simulink model "CardioVascularSystem"  (R2021b)
settings: Solver=daessc  StartTime=0.0  StopTime=Tend  MaxStep=0.6  RelTol=1e-3  AbsTol=1e-3
undefined symbols (not defined in the file): EsL, EsR, PipL, PipR, R1, R2, R3_fix, R4, R5, R6, R7, R8, RL, RR, tc, ts
libraries: fl_lib x54, nesl_utility x23, ee_lib x4, SignalEditorBlockLib x1
settings Model: Creator=mnord  LastModifiedBy=mnord
settings SolverCC: ZeroCrossAlgorithm=Adaptive  AlgebraicLoopSolver=TrustRegion
settings DebuggingCC: MaxConsecutiveZCsMsg=warning  IgnoredZcDiagnostic=none  SymbolicDimsDataTypeCodeGenerationDiagnostic=none  SFMachineParentedDataDiag=warning
settings SFSimCC: CustomCodeUndefinedFunction=UseInterfaceOnly
settings SimscapeCC: SimscapeLogType=all  SimscapeLogSimulationStatistics=on  SimscapeLogDataHistory=10000

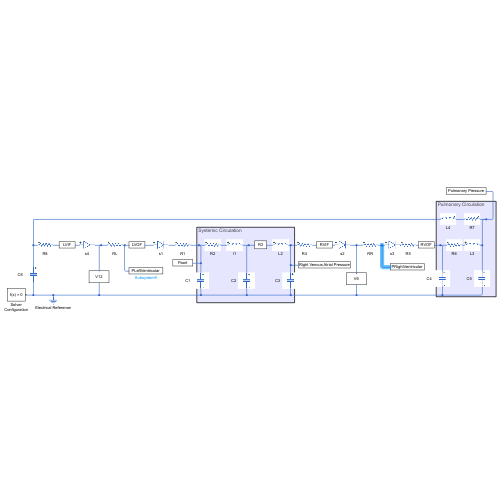
[thumbnail: Simulink's stored preview of the top-level diagram]
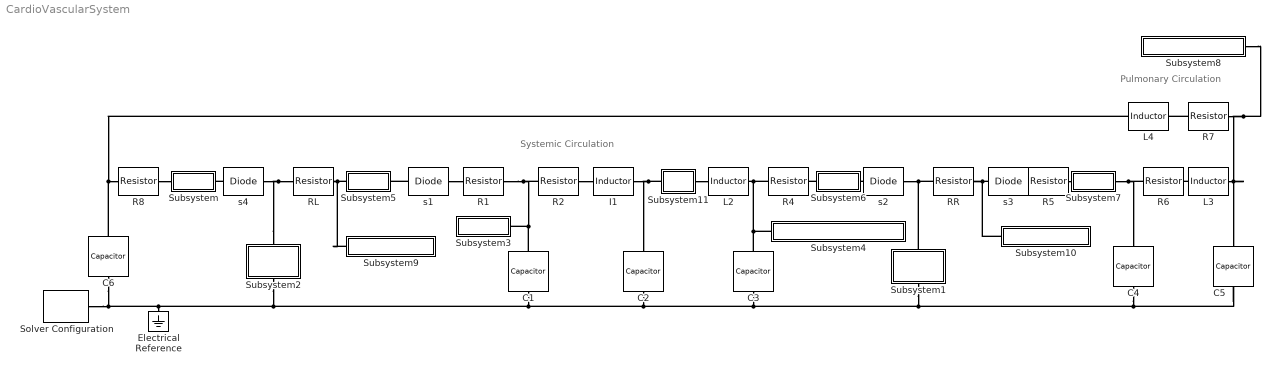
== system CardioVascularSystem ==
  note: Pulmonary Circulation
  note: Systemic Circulation
  C1 : fl_lib/Electrical/Electrical Elements/Capacitor  c=C1 F  r=capSerRes Ohm  g=0 1/Ohm  i_specify=off  i_priority=None  i=0 A  i_nominal_specify=off  i_nominal_unit=A  i_nominal_value=1  v_specify=off  v_priority=High  v=X10 V  v_nominal_specify=off  v_nominal_unit=V  v_nominal_value=1  vc_specify=on  vc_priority=High  vc=X10 V  vc_nominal_specify=off  vc_nominal_unit=V  vc_nominal_value=1
  C2 : fl_lib/Electrical/Electrical Elements/Capacitor  c=C2 F  r=capSerRes Ohm  g=0 1/Ohm  i_specify=off  i_priority=None  i=0 A  i_nominal_specify=off  i_nominal_unit=A  i_nominal_value=1  v_specify=off  v_priority=High  v=X30 V  v_nominal_specify=off  v_nominal_unit=V  v_nominal_value=1  vc_specify=on  vc_priority=High  vc=X30 V  vc_nominal_specify=off  vc_nominal_unit=V  vc_nominal_value=1
  C3 : fl_lib/Electrical/Electrical Elements/Capacitor  c=C3 F  r=capSerRes Ohm  g=0 1/Ohm  i_specify=off  i_priority=None  i=0 A  i_nominal_specify=off  i_nominal_unit=A  i_nominal_value=1  v_specify=off  v_priority=High  v=X50 V  v_nominal_specify=off  v_nominal_unit=V  v_nominal_value=1  vc_specify=on  vc_priority=High  vc=X50 V  vc_nominal_specify=off  vc_nominal_unit=V  vc_nominal_value=1
  C4 : fl_lib/Electrical/Electrical Elements/Capacitor  c=C4 F  r=capSerRes Ohm  g=0 1/Ohm  i_specify=off  i_priority=None  i=0 A  i_nominal_specify=off  i_nominal_unit=A  i_nominal_value=1  v_specify=off  v_priority=High  v=X70 V  v_nominal_specify=off  v_nominal_unit=V  v_nominal_value=1  vc_specify=on  vc_priority=High  vc=X70 V  vc_nominal_specify=off  vc_nominal_unit=V  vc_nominal_value=1
  C5 : fl_lib/Electrical/Electrical Elements/Capacitor  c=C5 F  r=capSerRes Ohm  g=0 1/Ohm  i_specify=off  i_priority=None  i=0 A  i_nominal_specify=off  i_nominal_unit=A  i_nominal_value=1  v_specify=off  v_priority=High  v=X90 V  v_nominal_specify=off  v_nominal_unit=V  v_nominal_value=1  vc_specify=on  vc_priority=High  vc=X90 V  vc_nominal_specify=off  vc_nominal_unit=V  vc_nominal_value=1
  C6 : fl_lib/Electrical/Electrical Elements/Capacitor  c=C6 F  r=capSerRes Ohm  g=0 1/Ohm  i_specify=off  i_priority=None  i=0 A  i_nominal_specify=off  i_nominal_unit=A  i_nominal_value=1  v_specify=off  v_priority=High  v=X110 V  v_nominal_specify=off  v_nominal_unit=V  v_nominal_value=1  vc_specify=on  vc_priority=High  vc=X110 V  vc_nominal_specify=off  vc_nominal_unit=V  vc_nominal_value=1
  Electrical Reference : fl_lib/Electrical/Electrical Elements/Electrical Reference
  I1 : ee_lib/Passive/Inductor  l=L1 H  L_tol=20  enable_L_tol=0  tol_distribution=1  nSigma=4  r=0 Ohm  g=1e-9 1/Ohm  enable_operating_limits=0  operating_limit_action=2  max_working_current=1 A  power_rating=1 W  enable_faults=0  fault_action=1  lambdaPercent=50  k_faulted=0.9999  turnsShort=0  openCct=0  groundShort=0  groundShortG=0 1/Ohm  tau_fault=1e-3 s  enable_temporal_fault=0  t_fault=1 s  enable_behavioral_fault=0  max_permissible_voltage=100 V  n_fail_on_voltage=1  max_permissible_current=1 A  t_fail_on_current=1 s  i_L_specify=on  i_L_priority=High  i_L=X20 A  i_L_nominal_specify=off  i_L_nominal_unit=A  i_L_nominal_value=1
  L2 : ee_lib/Passive/Inductor  l=L2 H  L_tol=20  enable_L_tol=0  tol_distribution=1  nSigma=4  r=0 Ohm  g=1e-9 1/Ohm  enable_operating_limits=0  operating_limit_action=2  max_working_current=1 A  power_rating=1 W  enable_faults=0  fault_action=1  lambdaPercent=50  k_faulted=0.9999  turnsShort=0  openCct=0  groundShort=0  groundShortG=0 1/Ohm  tau_fault=1e-3 s  enable_temporal_fault=0  t_fault=1 s  enable_behavioral_fault=0  max_permissible_voltage=100 V  n_fail_on_voltage=1  max_permissible_current=1 A  t_fail_on_current=1 s  i_L_specify=on  i_L_priority=High  i_L=X40 A  i_L_nominal_specify=off  i_L_nominal_unit=A  i_L_nominal_value=1
  L3 : ee_lib/Passive/Inductor  l=L3 H  L_tol=20  enable_L_tol=0  tol_distribution=1  nSigma=4  r=0 Ohm  g=1e-9 1/Ohm  enable_operating_limits=0  operating_limit_action=2  max_working_current=1 A  power_rating=1 W  enable_faults=0  fault_action=1  lambdaPercent=50  k_faulted=0.9999  turnsShort=0  openCct=0  groundShort=0  groundShortG=0 1/Ohm  tau_fault=1e-3 s  enable_temporal_fault=0  t_fault=1 s  enable_behavioral_fault=0  max_permissible_voltage=100 V  n_fail_on_voltage=1  max_permissible_current=1 A  t_fail_on_current=1 s  i_L_specify=on  i_L_priority=High  i_L=X80 A  i_L_nominal_specify=off  i_L_nominal_unit=A  i_L_nominal_value=1
  L4 : ee_lib/Passive/Inductor  l=L4 H  L_tol=20  enable_L_tol=0  tol_distribution=1  nSigma=4  r=0 Ohm  g=1e-9 1/Ohm  enable_operating_limits=0  operating_limit_action=2  max_working_current=1 A  power_rating=1 W  enable_faults=0  fault_action=1  lambdaPercent=50  k_faulted=0.9999  turnsShort=0  openCct=0  groundShort=0  groundShortG=0 1/Ohm  tau_fault=1e-3 s  enable_temporal_fault=0  t_fault=1 s  enable_behavioral_fault=0  max_permissible_voltage=100 V  n_fail_on_voltage=1  max_permissible_current=1 A  t_fail_on_current=1 s  i_L_specify=on  i_L_priority=High  i_L=X100 A  i_L_nominal_specify=off  i_L_nominal_unit=A  i_L_nominal_value=1
  R1 : fl_lib/Electrical/Electrical Elements/Resistor  R=R1 Ohm  i_specify=off  i_priority=None  i=0 A  i_nominal_specify=off  i_nominal_unit=A  i_nominal_value=1  v_specify=off  v_priority=None  v=0 V  v_nominal_specify=off  v_nominal_unit=V  v_nominal_value=1
  R2 : fl_lib/Electrical/Electrical Elements/Resistor  R=R2 Ohm  i_specify=off  i_priority=None  i=0 A  i_nominal_specify=off  i_nominal_unit=A  i_nominal_value=1  v_specify=off  v_priority=None  v=0 V  v_nominal_specify=off  v_nominal_unit=V  v_nominal_value=1
  R4 : fl_lib/Electrical/Electrical Elements/Resistor  R=R4 Ohm  i_specify=off  i_priority=None  i=0 A  i_nominal_specify=off  i_nominal_unit=A  i_nominal_value=1  v_specify=off  v_priority=None  v=0 V  v_nominal_specify=off  v_nominal_unit=V  v_nominal_value=1
  R5 : fl_lib/Electrical/Electrical Elements/Resistor  R=R5 Ohm  i_specify=off  i_priority=None  i=0 A  i_nominal_specify=off  i_nominal_unit=A  i_nominal_value=1  v_specify=off  v_priority=None  v=0 V  v_nominal_specify=off  v_nominal_unit=V  v_nominal_value=1
  R6 : fl_lib/Electrical/Electrical Elements/Resistor  R=R6 Ohm  i_specify=off  i_priority=None  i=0 A  i_nominal_specify=off  i_nominal_unit=A  i_nominal_value=1  v_specify=off  v_priority=None  v=0 V  v_nominal_specify=off  v_nominal_unit=V  v_nominal_value=1
  R7 : fl_lib/Electrical/Electrical Elements/Resistor  R=R7 Ohm  i_specify=off  i_priority=None  i=0 A  i_nominal_specify=off  i_nominal_unit=A  i_nominal_value=1  v_specify=off  v_priority=None  v=0 V  v_nominal_specify=off  v_nominal_unit=V  v_nominal_value=1
  R8 : fl_lib/Electrical/Electrical Elements/Resistor  R=R8 Ohm  i_specify=off  i_priority=None  i=0 A  i_nominal_specify=off  i_nominal_unit=A  i_nominal_value=1  v_specify=off  v_priority=None  v=0 V  v_nominal_specify=off  v_nominal_unit=V  v_nominal_value=1
  RL : fl_lib/Electrical/Electrical Elements/Resistor  R=RL Ohm  i_specify=off  i_priority=None  i=0 A  i_nominal_specify=off  i_nominal_unit=A  i_nominal_value=1  v_specify=off  v_priority=None  v=0 V  v_nominal_specify=off  v_nominal_unit=V  v_nominal_value=1
  RR : fl_lib/Electrical/Electrical Elements/Resistor  R=RR Ohm  i_specify=off  i_priority=None  i=0 A  i_nominal_specify=off  i_nominal_unit=A  i_nominal_value=1  v_specify=off  v_priority=None  v=0 V  v_nominal_specify=off  v_nominal_unit=V  v_nominal_value=1
  Solver Configuration : nesl_utility/Solver Configuration  PhysicalDomain=network_engine_domain  SubClassName=solver  LeftPortType=input  RightPortType=generic  Tones=[]  Harmonics=[]  SimulateNoise=off  Profile=off  UseLocalSampling=off  EnableSwitchedLinearOptims=on  FrequencyDomain=off  UseCCode=off  RelTol=0.001  AbsTol=1e-06  MinStep=1e-09  ToWorkspace=off  RevertToSquareIcSolve=off  NumHomotopyIterations=100  PhasorMode=off  PhasorModeNumHarmonics=1  DoDC=off  ResidualTolerance=1e-09  UseLocalSolver=off  LocalSolverChoice=NE_BACKWARD_EULER_ADVANCER  LocalSolverSampleTime=0.001  DoFixedCost=off  MaxNonlinIter=3  MaxModeIter=2  ComputeImpulses=off  ImpulseIterations=2  LinearAlgebra=auto  EquationFormulation=NE_TIME_EF  DelaysMemoryBudget=1024  AutomaticFiltering=on  FilteringTimeConstant=0.001  PartitionStorageMethod=AS_NEEDED  PartitionMemoryBudget=1024  PartitionMethod=ROBUST
      settings: SourceProductBaseCode=PW,SS
  Subsystem : Subsystem
      mask Display: disp('LVIF')
  Subsystem1 : Subsystem
      mask Display: disp('V6')
  Subsystem10 : Subsystem
      mask Display: disp('PRightVentricular')
  Subsystem11 : Subsystem
      mask Display: disp('R3')
  Subsystem2 : Subsystem
      mask Display: disp('V12')
  Subsystem3 : Subsystem
      mask Display: disp('Paort')
  Subsystem4 : Subsystem
      mask Display: disp('Right Venous Atrial Pressure')
  Subsystem5 : Subsystem
      mask Display: disp('LVOF')
  Subsystem6 : Subsystem
      mask Display: disp('RVIF')
  Subsystem7 : Subsystem
      mask Display: disp('RVOF')
  Subsystem8 : Subsystem
      mask Display: disp('Pulmonary Pressure')
  Subsystem9 : Subsystem
      mask Display: disp('PLeftVentricular')
  s{1..4} (4 alike) : fl_lib/Electrical/Electrical Elements/Diode  Vf=FwVolt V  Ron=onRes Ohm  Goff=1e-8 1/Ohm  i_specify=off  i_priority=None  i=0 A  i_nominal_specify=off  i_nominal_unit=A  i_nominal_value=1  v_specify=off  v_priority=None  v=0 V  v_nominal_specify=off  v_nominal_unit=V  v_nominal_value=1
  connections:
  C6/LConn1 -- R8/LConn1 -- L4/RConn1
  Subsystem11/RConn1 -- L2/LConn1
  I1/RConn1 -- Subsystem11/LConn1 -- C2/LConn1
  R4/LConn1 -- C3/LConn1 -- Subsystem4/LConn1 -- L2/RConn1
  L3/LConn1 -- R6/RConn1
  L3/RConn1 -- Subsystem8/LConn1 -- R7/LConn1 -- C5/LConn1
  R7/RConn1 -- L4/LConn1
  R8/RConn1 -- Subsystem/LConn1
  s4/LConn1 -- Subsystem/RConn1
  Subsystem3/LConn1 -- R2/LConn1 -- R1/RConn1 -- C1/LConn1
  Subsystem6/LConn1 -- R4/RConn1
  C6/RConn1 -- Solver Configuration/RConn1 -- Electrical Reference/LConn1 -- Subsystem2/RConn1 -- C5/RConn1 -- C4/RConn1 -- Subsystem1/RConn1 -- C3/RConn1 -- C2/RConn1 -- C1/RConn1
  RR/LConn1 -- Subsystem1/LConn1 -- s2/RConn1
  Subsystem2/LConn1 -- s4/RConn1 -- RL/LConn1
  s3/LConn1 -- Subsystem10/LConn1 -- RR/RConn1
  s3/RConn1 -- R5/LConn1
  R6/LConn1 -- C4/LConn1 -- Subsystem7/RConn1
  Subsystem5/LConn1 -- Subsystem9/LConn1 -- RL/RConn1
  s1/RConn1 -- R1/LConn1
  s2/LConn1 -- Subsystem6/RConn1
  R5/RConn1 -- Subsystem7/LConn1
  s1/LConn1 -- Subsystem5/RConn1
  R2/RConn1 -- I1/LConn1

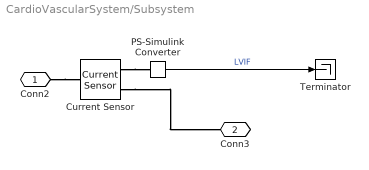
== system CardioVascularSystem/Subsystem ==
  Current Sensor : fl_lib/Electrical/Electrical Sensors/Current Sensor
  PS-Simulink Converter : nesl_utility/PS-Simulink Converter  PhysicalDomain=network_engine_domain  SubClassName=ps_output  LeftPortType=input  RightPortType=output  PseudoPeriodic=off  Frequencies=[]  Unit=inherit  AffineConversion=off
      settings: SourceProductBaseCode=PW,SS
  Terminator : Terminator
  Conn2 : PMIOPort  Side=Left
  Conn3 : PMIOPort  Port=2  Side=Right
  wires:
  PS-Simulink Converter/1 -> Terminator/1  "LVIF"
  connections:
  Conn2/RConn1 -- Current Sensor/LConn1
  Current Sensor/RConn2 -- Conn3/RConn1
  Current Sensor/RConn1 -- PS-Simulink Converter/LConn1

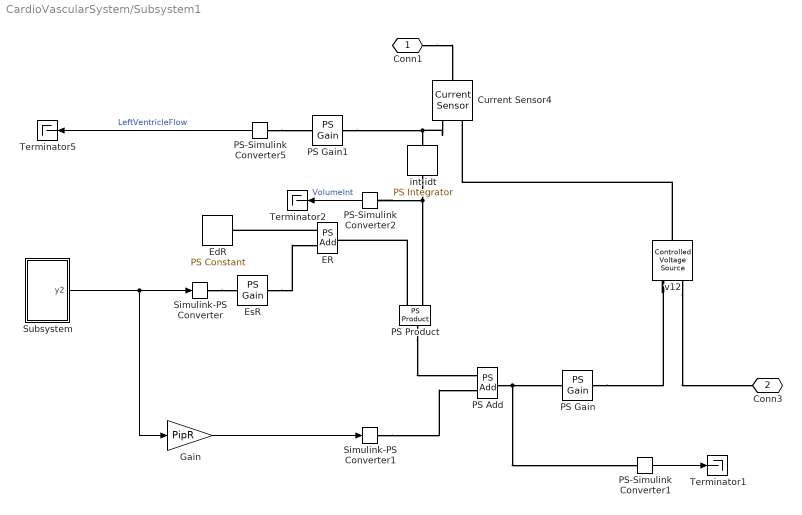
== system CardioVascularSystem/Subsystem1 ==
  Current Sensor4 : fl_lib/Electrical/Electrical Sensors/Current Sensor
  ER : fl_lib/Physical Signals/Functions/PS Add
  EdR : fl_lib/Physical Signals/Sources/PS Constant  constant=EdR
  EsR : fl_lib/Physical Signals/Functions/PS Gain  gain=EsR
  Gain : Gain  Gain=PipR
  PS Add : fl_lib/Physical Signals/Functions/PS Add
  PS Gain : fl_lib/Physical Signals/Functions/PS Gain  gain=1 V/s/A
  PS Gain1 : fl_lib/Physical Signals/Functions/PS Gain  gain=-1
  PS Product : fl_lib/Physical Signals/Functions/PS Product
  PS-Simulink Converter1 : nesl_utility/PS-Simulink Converter  PhysicalDomain=network_engine_domain  SubClassName=ps_output  LeftPortType=input  RightPortType=output  PseudoPeriodic=off  Frequencies=[]  Unit=inherit  AffineConversion=off
      settings: SourceProductBaseCode=PW,SS
  PS-Simulink Converter2 : nesl_utility/PS-Simulink Converter  PhysicalDomain=network_engine_domain  SubClassName=ps_output  LeftPortType=input  RightPortType=output  PseudoPeriodic=off  Frequencies=[]  Unit=inherit  AffineConversion=off
      settings: SourceProductBaseCode=PW,SS
  PS-Simulink Converter5 : nesl_utility/PS-Simulink Converter  PhysicalDomain=network_engine_domain  SubClassName=ps_output  LeftPortType=input  RightPortType=output  PseudoPeriodic=off  Frequencies=[]  Unit=inherit  AffineConversion=off
      settings: SourceProductBaseCode=PW,SS
  Simulink-PS Converter : nesl_utility/Simulink-PS Converter  PhysicalDomain=network_engine_domain  SubClassName=ps_input  LeftPortType=input  RightPortType=output  PseudoPeriodic=off  Frequencies=[]  NoiseDistribution=none  NoiseParameters=[]  Unit=1  AffineConversion=off  FilteringAndDerivatives=provide  SimscapeFilterOrder=1  InputFilterTimeConstant=0.001  UdotUserProvided=0
      settings: SourceProductBaseCode=PW,SS
  Simulink-PS Converter1 : nesl_utility/Simulink-PS Converter  PhysicalDomain=network_engine_domain  SubClassName=ps_input  LeftPortType=input  RightPortType=output  PseudoPeriodic=off  Frequencies=[]  NoiseDistribution=none  NoiseParameters=[]  Unit=A*s  AffineConversion=off  FilteringAndDerivatives=provide  SimscapeFilterOrder=1  InputFilterTimeConstant=0.001  UdotUserProvided=0
      settings: SourceProductBaseCode=PW,SS
  Subsystem : Subsystem
  Terminator1 : Terminator
  Terminator2 : Terminator
  Terminator5 : Terminator
  int idt : fl_lib/Physical Signals/Linear Operators/PS Integrator  reset_method=foundation.enum.IntegratorResetSpec.None  initial_condition_spec=foundation.enum.IntegratorICSpec.Internal  x0=X60 A*s
      settings: SourceProductBaseCode=SS
  v12 : fl_lib/Electrical/Electrical Sources/Controlled Voltage Source
  Conn1 : PMIOPort  Side=Left
  Conn3 : PMIOPort  Port=2  Side=Right
  wires:
  PS-Simulink Converter1/1 -> Terminator1/1
  Gain/1 -> Simulink-PS Converter1/1
  PS-Simulink Converter2/1 -> Terminator2/1  "VolumeInt"
  Subsystem/1(y2) -> Gain/1, Simulink-PS Converter/1
  PS-Simulink Converter5/1 -> Terminator5/1  "LeftVentricleFlow"
  connections:
  PS Add/RConn1 -- PS-Simulink Converter1/LConn1 -- PS Gain/LConn1
  PS-Simulink Converter2/LConn1 -- PS Product/LConn1 -- int idt/RConn1
  PS Product/RConn1 -- PS Add/LConn1
  v12/LConn1 -- Current Sensor4/RConn2
  ER/LConn1 -- EdR/RConn1
  Simulink-PS Converter1/RConn1 -- PS Add/LConn2
  EsR/RConn1 -- ER/LConn2
  PS Product/LConn2 -- ER/RConn1
  v12/RConn2 -- Conn3/RConn1
  Conn1/RConn1 -- Current Sensor4/LConn1
  Current Sensor4/RConn1 -- PS Gain1/LConn1 -- int idt/LConn1
  Simulink-PS Converter/RConn1 -- EsR/LConn1
  PS Gain/RConn1 -- v12/RConn1
  PS-Simulink Converter5/LConn1 -- PS Gain1/RConn1

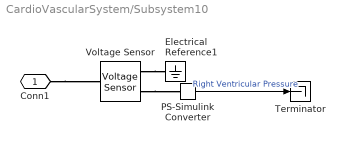
== system CardioVascularSystem/Subsystem10 ==
  Electrical Reference1 : fl_lib/Electrical/Electrical Elements/Electrical Reference
  PS-Simulink Converter : nesl_utility/PS-Simulink Converter  PhysicalDomain=network_engine_domain  SubClassName=ps_output  LeftPortType=input  RightPortType=output  PseudoPeriodic=off  Frequencies=[]  Unit=inherit  AffineConversion=off
      settings: SourceProductBaseCode=PW,SS
  Terminator : Terminator
  Voltage Sensor : fl_lib/Electrical/Electrical Sensors/Voltage Sensor
  Conn1 : PMIOPort  Side=Left
  wires:
  PS-Simulink Converter/1 -> Terminator/1  "Right Ventricular Pressure"
  connections:
  Conn1/RConn1 -- Voltage Sensor/LConn1
  Voltage Sensor/RConn2 -- Electrical Reference1/LConn1
  Voltage Sensor/RConn1 -- PS-Simulink Converter/LConn1

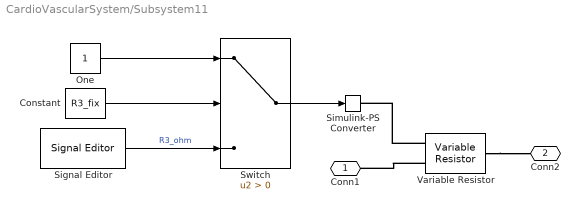
== system CardioVascularSystem/Subsystem11 ==
  Constant : Constant  Value=R3_fix
  One : Constant  OutDataTypeStr=Inherit: Inherit via back propagation
  Signal Editor : SignalEditorBlockLib/Signal Editor  FileName=R3_Values.mat  ActiveScenario=Scenario  ActiveSignal=Signal 1  IsBus=off  OutputBusObjectStr=Bus: BusObject  SampleTime=0  Interpolate=off  ZeroCross=off  OutputAfterFinalValue=Holding final value  Unit=inherit  PreserveSignalName=on
  Simulink-PS Converter : nesl_utility/Simulink-PS Converter  PhysicalDomain=network_engine_domain  SubClassName=ps_input  LeftPortType=input  RightPortType=output  PseudoPeriodic=off  Frequencies=[]  NoiseDistribution=none  NoiseParameters=[]  Unit=1  AffineConversion=off  FilteringAndDerivatives=filter  SimscapeFilterOrder=1  InputFilterTimeConstant=0.1  UdotUserProvided=0
      settings: SourceProductBaseCode=PW,SS
  Switch : Switch  Criteria=u2 > Threshold
  Variable Resistor : fl_lib/Electrical/Electrical Elements/Variable Resistor  Rmin=0 Ohm  i_specify=off  i_priority=None  i=0 A  i_nominal_specify=off  i_nominal_unit=A  i_nominal_value=1  v_specify=off  v_priority=None  v=0 V  v_nominal_specify=off  v_nominal_unit=V  v_nominal_value=1
  Conn1 : PMIOPort  Side=Left
  Conn2 : PMIOPort  Port=2  Side=Right
  wires:
  Signal Editor/1 -> Switch/3  "R3_ohm"
  One/1 -> Switch/1
  Constant/1 -> Switch/2
  Switch/1 -> Simulink-PS Converter/1
  connections:
  Variable Resistor/LConn1 -- Simulink-PS Converter/RConn1
  Variable Resistor/LConn2 -- Conn1/RConn1
  Variable Resistor/RConn1 -- Conn2/RConn1

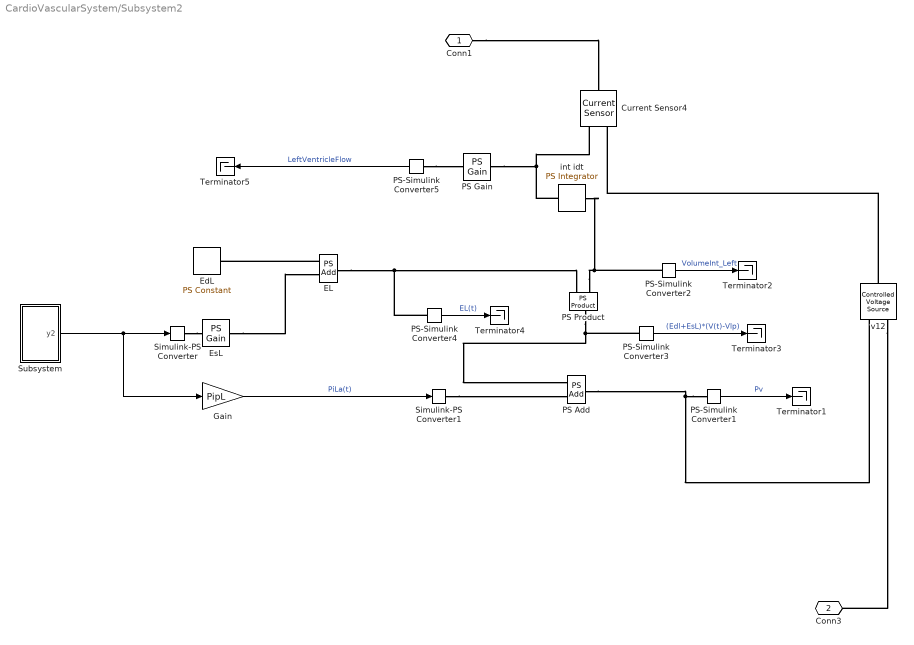
== system CardioVascularSystem/Subsystem2 ==
  Current Sensor4 : fl_lib/Electrical/Electrical Sensors/Current Sensor
  EL : fl_lib/Physical Signals/Functions/PS Add
  EdL : fl_lib/Physical Signals/Sources/PS Constant  constant=EdL V/A/s
  EsL : fl_lib/Physical Signals/Functions/PS Gain  gain=EsL
  Gain : Gain  Gain=PipL
  PS Add : fl_lib/Physical Signals/Functions/PS Add
  PS Gain : fl_lib/Physical Signals/Functions/PS Gain  gain=-1
  PS Product : fl_lib/Physical Signals/Functions/PS Product
  PS-Simulink Converter{1..5} (5 alike) : nesl_utility/PS-Simulink Converter  PhysicalDomain=network_engine_domain  SubClassName=ps_output  LeftPortType=input  RightPortType=output  PseudoPeriodic=off  Frequencies=[]  Unit=inherit  AffineConversion=off
      settings: SourceProductBaseCode=PW,SS
  Simulink-PS Converter : nesl_utility/Simulink-PS Converter  PhysicalDomain=network_engine_domain  SubClassName=ps_input  LeftPortType=input  RightPortType=output  PseudoPeriodic=off  Frequencies=[]  NoiseDistribution=none  NoiseParameters=[]  Unit=V/A/s  AffineConversion=off  FilteringAndDerivatives=provide  SimscapeFilterOrder=1  InputFilterTimeConstant=0.001  UdotUserProvided=0
      settings: SourceProductBaseCode=PW,SS
  Simulink-PS Converter1 : nesl_utility/Simulink-PS Converter  PhysicalDomain=network_engine_domain  SubClassName=ps_input  LeftPortType=input  RightPortType=output  PseudoPeriodic=off  Frequencies=[]  NoiseDistribution=none  NoiseParameters=[]  Unit=V  AffineConversion=off  FilteringAndDerivatives=provide  SimscapeFilterOrder=1  InputFilterTimeConstant=0.001  UdotUserProvided=0
      settings: SourceProductBaseCode=PW,SS
  Subsystem : Subsystem
  Terminator{1..5} (5 alike) : Terminator
  int idt : fl_lib/Physical Signals/Linear Operators/PS Integrator  reset_method=foundation.enum.IntegratorResetSpec.None  initial_condition_spec=foundation.enum.IntegratorICSpec.Internal  x0=X120 A*s
      settings: SourceProductBaseCode=SS
  v12 : fl_lib/Electrical/Electrical Sources/Controlled Voltage Source
  Conn1 : PMIOPort  Side=Left
  Conn3 : PMIOPort  Port=2  Side=Right
  wires:
  Gain/1 -> Simulink-PS Converter1/1  "PiLa(t)"
  Subsystem/1(y2) -> Gain/1, Simulink-PS Converter/1
  PS-Simulink Converter1/1 -> Terminator1/1  "Pv"
  PS-Simulink Converter2/1 -> Terminator2/1  "VolumeInt_Left"
  PS-Simulink Converter3/1 -> Terminator3/1  "(Edl+EsL)*(V(t)-Vlp)"
  PS-Simulink Converter4/1 -> Terminator4/1  "EL(t)"
  PS-Simulink Converter5/1 -> Terminator5/1  "LeftVentricleFlow"
  connections:
  PS Product/LConn1 -- int idt/RConn1 -- PS-Simulink Converter2/LConn1
  EL/LConn1 -- EdL/RConn1
  EsL/RConn1 -- EL/LConn2
  Simulink-PS Converter1/RConn1 -- PS Add/LConn2
  Simulink-PS Converter/RConn1 -- EsL/LConn1
  v12/RConn2 -- Conn3/RConn1
  int idt/LConn1 -- PS Gain/LConn1 -- Current Sensor4/RConn1
  Conn1/RConn1 -- Current Sensor4/LConn1
  EL/RConn1 -- PS-Simulink Converter4/LConn1 -- PS Product/LConn2
  PS-Simulink Converter1/LConn1 -- v12/RConn1 -- PS Add/RConn1
  v12/LConn1 -- Current Sensor4/RConn2
  PS Product/RConn1 -- PS Add/LConn1 -- PS-Simulink Converter3/LConn1
  PS-Simulink Converter5/LConn1 -- PS Gain/RConn1

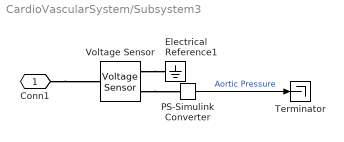
== system CardioVascularSystem/Subsystem3 ==
  Electrical Reference1 : fl_lib/Electrical/Electrical Elements/Electrical Reference
  PS-Simulink Converter : nesl_utility/PS-Simulink Converter  PhysicalDomain=network_engine_domain  SubClassName=ps_output  LeftPortType=input  RightPortType=output  PseudoPeriodic=off  Frequencies=[]  Unit=inherit  AffineConversion=off
      settings: SourceProductBaseCode=PW,SS
  Terminator : Terminator
  Voltage Sensor : fl_lib/Electrical/Electrical Sensors/Voltage Sensor
  Conn1 : PMIOPort  Side=Left
  wires:
  PS-Simulink Converter/1 -> Terminator/1  "Aortic Pressure"
  connections:
  Voltage Sensor/RConn1 -- PS-Simulink Converter/LConn1
  Voltage Sensor/RConn2 -- Electrical Reference1/LConn1
  Conn1/RConn1 -- Voltage Sensor/LConn1

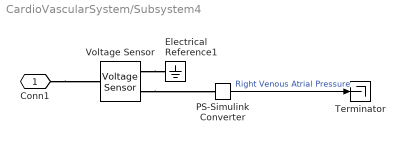
== system CardioVascularSystem/Subsystem4 ==
  Electrical Reference1 : fl_lib/Electrical/Electrical Elements/Electrical Reference
  PS-Simulink Converter : nesl_utility/PS-Simulink Converter  PhysicalDomain=network_engine_domain  SubClassName=ps_output  LeftPortType=input  RightPortType=output  PseudoPeriodic=off  Frequencies=[]  Unit=inherit  AffineConversion=off
      settings: SourceProductBaseCode=PW,SS
  Terminator : Terminator
  Voltage Sensor : fl_lib/Electrical/Electrical Sensors/Voltage Sensor
  Conn1 : PMIOPort  Side=Left
  wires:
  PS-Simulink Converter/1 -> Terminator/1  "Right Venous Atrial Pressure"
  connections:
  Conn1/RConn1 -- Voltage Sensor/LConn1
  Voltage Sensor/RConn2 -- Electrical Reference1/LConn1
  Voltage Sensor/RConn1 -- PS-Simulink Converter/LConn1

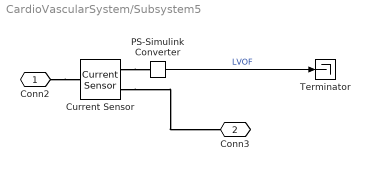
== system CardioVascularSystem/Subsystem5 ==
  Current Sensor : fl_lib/Electrical/Electrical Sensors/Current Sensor
  PS-Simulink Converter : nesl_utility/PS-Simulink Converter  PhysicalDomain=network_engine_domain  SubClassName=ps_output  LeftPortType=input  RightPortType=output  PseudoPeriodic=off  Frequencies=[]  Unit=inherit  AffineConversion=off
      settings: SourceProductBaseCode=PW,SS
  Terminator : Terminator
  Conn2 : PMIOPort  Side=Left
  Conn3 : PMIOPort  Port=2  Side=Right
  wires:
  PS-Simulink Converter/1 -> Terminator/1  "LVOF"
  connections:
  Conn2/RConn1 -- Current Sensor/LConn1
  Current Sensor/RConn2 -- Conn3/RConn1
  Current Sensor/RConn1 -- PS-Simulink Converter/LConn1

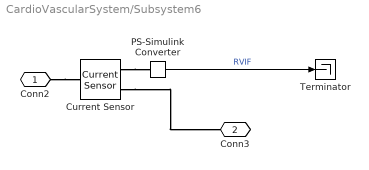
== system CardioVascularSystem/Subsystem6 ==
  Current Sensor : fl_lib/Electrical/Electrical Sensors/Current Sensor
  PS-Simulink Converter : nesl_utility/PS-Simulink Converter  PhysicalDomain=network_engine_domain  SubClassName=ps_output  LeftPortType=input  RightPortType=output  PseudoPeriodic=off  Frequencies=[]  Unit=inherit  AffineConversion=off
      settings: SourceProductBaseCode=PW,SS
  Terminator : Terminator
  Conn2 : PMIOPort  Side=Left
  Conn3 : PMIOPort  Port=2  Side=Right
  wires:
  PS-Simulink Converter/1 -> Terminator/1  "RVIF"
  connections:
  Current Sensor/RConn1 -- PS-Simulink Converter/LConn1
  Current Sensor/RConn2 -- Conn3/RConn1
  Conn2/RConn1 -- Current Sensor/LConn1

== system CardioVascularSystem/Subsystem7 ==
  Current Sensor : fl_lib/Electrical/Electrical Sensors/Current Sensor
  PS-Simulink Converter : nesl_utility/PS-Simulink Converter  PhysicalDomain=network_engine_domain  SubClassName=ps_output  LeftPortType=input  RightPortType=output  PseudoPeriodic=off  Frequencies=[]  Unit=inherit  AffineConversion=off
      settings: SourceProductBaseCode=PW,SS
  Terminator : Terminator
  Conn2 : PMIOPort  Side=Left
  Conn3 : PMIOPort  Port=2  Side=Right
  wires:
  PS-Simulink Converter/1 -> Terminator/1  "RVOF"
  connections:
  Conn2/RConn1 -- Current Sensor/LConn1
  Current Sensor/RConn2 -- Conn3/RConn1
  Current Sensor/RConn1 -- PS-Simulink Converter/LConn1

== system CardioVascularSystem/Subsystem8 ==
  Electrical Reference1 : fl_lib/Electrical/Electrical Elements/Electrical Reference
  PS-Simulink Converter : nesl_utility/PS-Simulink Converter  PhysicalDomain=network_engine_domain  SubClassName=ps_output  LeftPortType=input  RightPortType=output  PseudoPeriodic=off  Frequencies=[]  Unit=inherit  AffineConversion=off
      settings: SourceProductBaseCode=PW,SS
  Terminator : Terminator
  Voltage Sensor : fl_lib/Electrical/Electrical Sensors/Voltage Sensor
  Conn1 : PMIOPort  Side=Left
  wires:
  PS-Simulink Converter/1 -> Terminator/1  "Pulmonary Pressure"
  connections:
  Conn1/RConn1 -- Voltage Sensor/LConn1
  Voltage Sensor/RConn2 -- Electrical Reference1/LConn1
  Voltage Sensor/RConn1 -- PS-Simulink Converter/LConn1

== system CardioVascularSystem/Subsystem9 ==
  Electrical Reference1 : fl_lib/Electrical/Electrical Elements/Electrical Reference
  PS-Simulink Converter : nesl_utility/PS-Simulink Converter  PhysicalDomain=network_engine_domain  SubClassName=ps_output  LeftPortType=input  RightPortType=output  PseudoPeriodic=off  Frequencies=[]  Unit=inherit  AffineConversion=off
      settings: SourceProductBaseCode=PW,SS
  Terminator : Terminator
  Voltage Sensor : fl_lib/Electrical/Electrical Sensors/Voltage Sensor
  Conn1 : PMIOPort  Side=Left
  wires:
  PS-Simulink Converter/1 -> Terminator/1  "Left Ventricular Pressure"
  connections:
  Conn1/RConn1 -- Voltage Sensor/LConn1
  Voltage Sensor/RConn2 -- Electrical Reference1/LConn1
  Voltage Sensor/RConn1 -- PS-Simulink Converter/LConn1

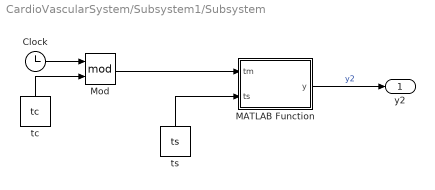
== system CardioVascularSystem/Subsystem1/Subsystem ==
  Clock : Clock
  MATLAB Function : MATLAB Function  TreatAsAtomicUnit=on
  Mod : Math  Operator=mod  SaturateOnIntegerOverflow=on
  tc : Constant  Value=tc
  ts : Constant  Value=ts
  y2 : Outport
  wires:
  Clock/1 -> Mod/1
  Mod/1 -> MATLAB Function/1(tm)
  MATLAB Function/1(y) -> y2/1  "y2"
  ts/1 -> MATLAB Function/2(ts)
  tc/1 -> Mod/2

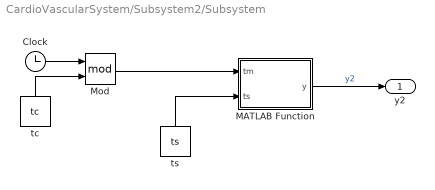
== system CardioVascularSystem/Subsystem2/Subsystem ==
  Clock : Clock
  MATLAB Function : MATLAB Function  TreatAsAtomicUnit=on
  Mod : Math  Operator=mod  SaturateOnIntegerOverflow=on
  tc : Constant  Value=tc
  ts : Constant  Value=ts
  y2 : Outport
  wires:
  Clock/1 -> Mod/1
  Mod/1 -> MATLAB Function/1(tm)
  MATLAB Function/1(y) -> y2/1  "y2"
  ts/1 -> MATLAB Function/2(ts)
  tc/1 -> Mod/2

== matlab function CardioVascularSystem/Subsystem2/Subsystem/MATLAB Function ==
  data: tm input; y output; ts input
function y = fcn(tm, ts)

if(tm< ts)
    y = (1-cos(2*pi*tm/ts)) * 0.5;
else
    y = 0;
end

== matlab function CardioVascularSystem/Subsystem1/Subsystem/MATLAB Function ==
  data: tm input; y output; ts input
function y = fcn(tm, ts)

if(tm< ts)
    y = (1-cos(2*pi*tm/ts)) * 0.5;
else
    y = 0;
end
